simulink model "AEBWithHighFidelityDynamicsTestBench"  (R2023b)
settings: Solver=ode23tb  StartTime=0  StopTime=30  FixedStep=Ts  MaxStep=Ts  RelTol=1e-1  AbsTol=5e-3
PostLoadFcn:
  | helperSLAEBWithHighFidelityDynamicsSetup();
  | load(fullfile(matlabroot,'toolbox','driving','drivingdata','rrScenarioSimTypes.mat'));
values from neighbouring files (symbols this model uses):
  actorProfiles = helperGetActorProfiles(world.actors,OriginOffset="RearAxleCenter")    [helperSLAEBWithHighFidelityDynamicsSetup.m]
  egoActorID = id    [helperSLAEBWithHighFidelityDynamicsSetup.m]
  egoVehDyn = egoVehicleDynamicsParams(egoInitialPose, actorProfiles(egoActorID))    [helperSLAEBWithHighFidelityDynamicsSetup.m]
  m = 1575    [helperSLAEBWithHighFidelityDynamicsSetup.m]
  Ts = 0.05    [helperSLAEBWithHighFidelityDynamicsSetup.m]
  vehSim3D = repmat(     struct(         'Length', 0,         'RearOverhang', 0,         'InitialPos',[0 0 0],         'InitialRot',[0 0 0]),     numVehicles,1)    [helperSLAEBWithHighFidelityDynamicsSetup.m]
undefined symbols (not defined in the file or in its folder): Defined, Ego, Lane, maxNumActors, n, radarParams, User, v_set
libraries: roadrunnerscenario x5, simulink x4, sim3dautolib x3, sim3dprobsensorlib x2, sim3dlib x1, sim3dgroundtruthsensorlib x1, drivingsim3d x1, drivingscenarioandsensors x1
CloseFcn:
  | helperSLAEBWithHighFidelityDynamicsCleanup
settings Model: SILPILSystemUnderTest=refmodels  SnapshotInterval=5  PacingRate=0.220000  Creator=The MathWorks, Inc.  LastModifiedBy=user
settings SolverCC: MaxConsecutiveZCs=1  MaxConsecutiveMinStep=2  ZeroCrossAlgorithm=Adaptive  AlgebraicLoopSolver=TrustRegion  SolverResetMethod=Robust  MinimalZcImpactIntegration=on  MaxZcPerStep=1
settings DataIOCC: SaveOutput=off  DSMLogging=off  SaveTime=off  ReturnWorkspaceOutputs=off  Refine=3
settings OptimizationCC: DefaultParameterBehavior=Inlined  InlineInvariantSignals=on  ReuseModelBlockBuffer=off  PassReuseOutputArgsAs=Individual arguments  ZeroExternalMemoryAtStartup=off  OptimizeBlockOrder=speed  EfficientTunableParamExpr=on
settings DebuggingCC: IgnoredZcDiagnostic=none  ParameterTunabilityLossMsg=error  UnconnectedInputMsg=warning  UnconnectedOutputMsg=warning  UnconnectedLineMsg=warning  PregeneratedLibrarySubsystemCodeDiagnostic=none  ArithmeticOperatorsInVariantConditions=warning
settings HardwareCC: ProdLongLongMode=on
settings ModelReferenceCC: EnableRefExpFcnMdlSchedulingChecks=on  ModelReferenceNumInstancesAllowed=Single  PropagateVarSize=Only when enabling
settings SFSimCC: SimUseLocalCustomCode=off  CustomCodeUndefinedFunction=UseInterfaceOnly
settings RTWCC: Description=Embedded Coder  SystemTargetFile=ert.tlc  TemplateMakefile=ert_default_tmf  GenerateReport=on  RTWUseLocalCustomCode=off  Toolchain=MinGW64 | CMake/gmake (64-bit Windows)  BuildConfiguration=Release  IncludeHyperlinkInReport=on  LaunchReport=on  GenerateTraceInfo=on  GenerateTraceReport=on  GenerateTraceReportSl=on  GenerateTraceReportSf=on  GenerateTraceReportEml=on  GenerateCodeMetricsReport=on  DLArmComputeVersion=19.05
settings CodeAppCC: ForceParamTrailComments=on  IgnoreCustomStorageClasses=off  OperatorAnnotations=on  SimulinkDataObjDesc=on  SFDataObjDesc=on  CustomSymbolStrFcn=$N$M$F  InsertBlockDesc=on
settings ERTTargetCC: TargetLangStandard=C99 (ISO)  GenerateSampleERTMain=on  CombineSignalStateStructs=on  SuppressErrorStatus=on  InlinedParameterPlacement=NonHierarchical  RootIOFormat=Structure reference  RTWCAPISignals=on  ERTCustomFileTemplate=example_file_process.tlc

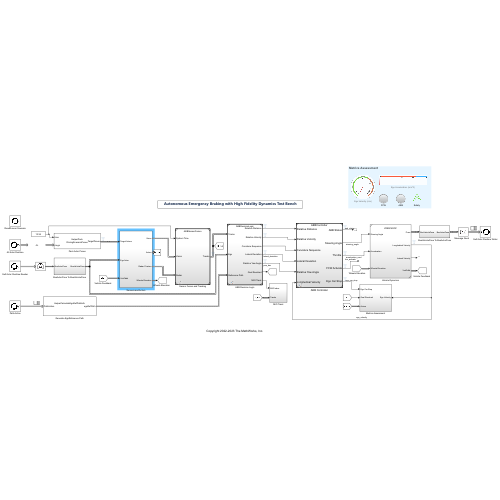
[thumbnail: Simulink's stored preview of the top-level diagram]
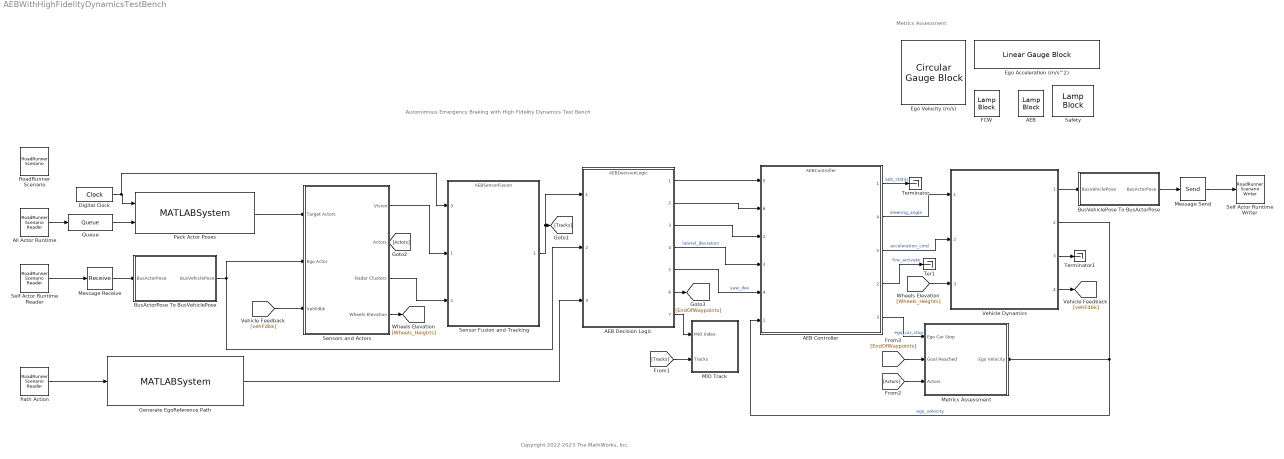
== system AEBWithHighFidelityDynamicsTestBench ==
  note: Copyright 2022-2023 The MathWorks, Inc.
  note: Autonomous Emergency Braking with High Fidelity Dynamics Test Bench
  note: Metrics Assessment
  AEB : LampBlock  LabelPosition=Hide
  AEB Controller : ModelReference  ModelNameDialog=AEBController.slx  SimulationMode=Normal  CodeInterface=Top model  ModelReferenceVersion=7.2
      settings: PortSchema="{\"entries\":[{\"content\":{\"sides\":[{\"content\":{\"connectorIds\":[\"In5\",\"In6\",\"In2\",\"In3\",\"In4\",\"In1\"]},\"type\":\"ConnectorPlacement.EquallySpacedRectSide\",\"uuid\":\"48eb62e1-c687-4ccc-af1d-5db323c86b02\"},{\"content\":{\"connectorIds\":[\"Out1\",\"Out4\",\"Out5\",\"Out2\",\"Out3\"],\"side\":\"RIGHT\"},\"type\":\"ConnectorPlacement.EquallySpacedRectSide\",\"uuid\":\"cf0b79c1-cc3c-4144-ab0a-ade48c99ebae\"},{\"content\":{\"connectorIds\":[],\"side\":\"TOP\"},\"type\":\"ConnectorPlacement.EquallySpacedRectSide\",\"uuid\":\"b5029296-17a7-4a3b-9030-50c7482e3f67\"}]},\"type\":\"ConnectorPlacement.EquallySpacedConnector\",\"uuid\":\"17fe6146-247b-40c2-bc98-b1cbe9fc8f16\"}],\"packageUris\":[\"http://schema.mathworks.com/mf0/Connector/R2020b\"],\"version\":\"1.0\"}"
  AEB Decision Logic : ModelReference  ModelNameDialog=AEBDecisionLogic.slx  SimulationMode=Normal  CodeInterface=Top model  ModelReferenceVersion=7.2
  All Actor Runtime : roadrunnerscenario/RoadRunner Scenario Reader  TopicCategory=Actor  ActorCategory=All Types  ActionType=Path Following  EventType=User-Defined  TopicType=Actor Pose (Driving Scenario compatible)  VehicleType=Vehicle Pose  UserDefinedAction=Action1  UserDefinedEvent=Event1  Filter=None  SensorTopic=Target Poses  LaneBoundaryOutputTopic=Ego-Lane  SensorID=1  SampleTime=Ts
  BusActorPose To BusVehiclePose : Subsystem
  BusVehiclePose To BusActorPose : Subsystem
  Digital Clock : DigitalClock  SampleTime=Ts
  Ego Acceleration (m/s^2) : LinearGaugeBlock  LabelPosition=Hide  ScaleMin=-9.8  ScaleMax=3  TickInterval=3
  Ego Velocity (m/s) : CircularGaugeBlock  LabelPosition=Hide  ScaleMax=25
  FCW : LampBlock  LabelPosition=Hide
  Generate EgoReference Path : MATLABSystem  InputPortMessageModes=m  System=HelperCalculateEgoRefPathInfo  EgoSpeed=v_set  SpaceResolution=DiscretizationDistance  DefaultEgoRefPath="Simulink.Bus.createMATLABStruct( \"BusEgoRefPath\" )"
      mask Type: HelperCalculateEgoRefPathInfo
      mask Display:
      | disp(['HelperCalculateEgoRefPathInfo' char(10) '' char(10) '']);
      | port_label('input',1,'PathAction');
      | port_label('output',1,'egoRefPath');
  MIO Track : Subsystem
  Message Receive : Receive  InputPortMessageModes=m  SampleTime=Ts
  "Message Send     " : Send  OutputPortMessageModes=m
  Metrics Assessment : Subsystem
      settings: PortSchema="{\"entries\":[{\"content\":{\"sides\":[{\"content\":{\"connectorIds\":[\"In1\",\"In2\",\"In3\"]},\"type\":\"ConnectorPlacement.EquallySpacedRectSide\",\"uuid\":\"d600d027-9714-4589-bd74-ff85c373770c\"},{\"content\":{\"connectorIds\":[\"In4\"],\"side\":\"RIGHT\"},\"type\":\"ConnectorPlacement.EquallySpacedRectSide\",\"uuid\":\"c68a0d3a-3a81-49cd-ba70-f2de3f1a882f\"},{\"content\":{\"connectorIds\":[],\"side\":\"TOP\"},\"type\":\"ConnectorPlacement.EquallySpacedRectSide\",\"uuid\":\"d9b15fac-7ed3-4474-96f3-d7b693286234\"},{\"content\":{\"connectorIds\":[],\"side\":\"BOTTOM\"},\"type\":\"ConnectorPlacement.EquallySpacedRectSide\",\"uuid\":\"00c5a332-b546-4dc5-aa31-259f1868ab67\"}]},\"type\":\"ConnectorPlacement.EquallySpacedConnector\",\"uuid\":\"e6d068d7-d2df-4de9-99aa-2a189a2c2730\"}],\"packageUris\":[\"http://schema.mathworks.com/mf0/Connector/R2020b\"],\"version\":\"1.0\"}"
  Pack Actor Poses : MATLABSystem  InputPortMessageModes=n,m  System=HelperPackDrivingScenarioPoses  EgoActorID=1  ActorProfiles=struct( 'ActorID', 1, 'ClassID', 1, 'Length', 4.7, 'Width', 1.8, 'Height', 1.4, 'OriginOffset', [ 0, 0, 0 ], 'FrontOverhang', 0, 'RearOverhang', 0, 'Wheelbase', 0, 'Color', [ 0, 0, 0 ] )  DefaultActorPoses="Simulink.Bus.createMATLABStruct( \"BusActors\" )"
      mask Type: HelperPackDrivingScenarioPoses
      mask Display:
      | disp(['HelperPack' char(10) 'DrivingScenarioPoses']);
      | port_label('input',1,'time');
      | port_label('input',2,'msgs');
      | port_label('output',1,'TargetPoses');
  Path Action : roadrunnerscenario/RoadRunner Scenario Reader  TopicCategory=Action  ActorCategory=All Types  ActionType=Path Following  EventType=User-Defined  TopicType=Actor Pose (Driving Scenario compatible)  VehicleType=Vehicle Specifications  UserDefinedAction=Action1  UserDefinedEvent=Event1  Filter=Self  SensorTopic=Target Poses  LaneBoundaryOutputTopic=Ego-Lane  SensorID=1  SampleTime=Ts
  Queue : Queue  InputPortMessageModes=m  OutputPortMessageModes=m  OverwriteOldest=on  Capacity=maxNumActors + 2
  RoadRunner Scenario : roadrunnerscenario/RoadRunner Scenario  UserDefinedActions={}  UserDefinedEvents={}
  Safety : LampBlock  LabelPosition=Hide  Icon=Hazards
  Self Actor Runtime Reader : roadrunnerscenario/RoadRunner Scenario Reader  TopicCategory=Actor  ActorCategory=All Types  ActionType=Path Following  EventType=User-Defined  TopicType=Actor Pose (Driving Scenario compatible)  VehicleType=Vehicle Specifications  UserDefinedAction=Action1  UserDefinedEvent=Event1  Filter=Self  SensorTopic=Target Poses  LaneBoundaryOutputTopic=Ego-Lane  SensorID=1  SampleTime=Ts
  Self Actor Runtime Writer : roadrunnerscenario/RoadRunner Scenario Writer  TopicCategory=Actor  ActorCategory=All Types  EventType=Action Complete  UserDefinedEvent=Event1  VehicleType=Vehicle Pose  TopicType=Actor Pose (Driving Scenario compatible)
  Sensor Fusion and Tracking : ModelReference  ModelNameDialog=AEBSensorFusion.slx  SimulationMode=Normal  CodeInterface=Top model  ModelReferenceVersion=7.2
      settings: PortSchema="{\"entries\":[{\"content\":{\"sides\":[{\"content\":{\"connectorIds\":[\"In3\",\"In1\",\"In2\"]},\"type\":\"ConnectorPlacement.EquallySpacedRectSide\",\"uuid\":\"d9651454-d0c0-4076-b933-d1c75ec1a64d\"},{\"content\":{\"connectorIds\":[\"Out1\"],\"side\":\"RIGHT\"},\"type\":\"ConnectorPlacement.EquallySpacedRectSide\",\"uuid\":\"0cfd8cd3-0315-45db-9435-2ff03149d1d1\"},{\"content\":{\"connectorIds\":[],\"side\":\"TOP\"},\"type\":\"ConnectorPlacement.EquallySpacedRectSide\",\"uuid\":\"cae0d945-b7aa-4a36-92d8-77152c4bc864\"}]},\"type\":\"ConnectorPlacement.EquallySpacedConnector\",\"uuid\":\"34f6be1b-6fa5-478f-9dd8-3c13b85e5ba6\"}],\"packageUris\":[\"http://schema.mathworks.com/mf0/Connector/R2020b\"],\"version\":\"1.0\"}"
  Sensors and Actors : Subsystem
  Ter1 : Terminator
  Terminator : Terminator
  Terminator1 : Terminator
  Vehicle Dynamics : Subsystem  ReferencedSubsystem=VDBS14DOF
  wires:
  AEB Controller/1 -> Terminator/1  "aeb_status"
  AEB Controller/2 -> Ter1/1  "fcw_activate"
  Vehicle Dynamics/2 -> Metrics Assessment/4(Ego Velocity), AEB Controller/1  "ego_velocity"
  [Actors] -> Metrics Assessment/3(Actors)
  [EndOfWaypoints] -> Metrics Assessment/2(Goal Reached)
  [Tracks] -> MIO Track/2(Tracks)
  AEB Controller/3 -> Metrics Assessment/1(Ego Car Stop)  "ego_car_stop"
  All Actor Runtime/1 -> Queue/1
  Queue/1 -> Pack Actor Poses/2
  Vehicle Dynamics/3 -> Terminator1/1
  Sensors and Actors/2(Actors) -> [Actors]
  Path Action/1 -> Generate EgoReference Path/1
  Pack Actor Poses/1 -> Sensors and Actors/1(Target Actors)
  AEB Controller/4 -> Vehicle Dynamics/1  "steering_angle"
  AEB Controller/5 -> Vehicle Dynamics/2  "acceleration_cmd"
  "Message Send     "/1 -> Self Actor Runtime Writer/1
  Sensors and Actors/4(Wheels Elevation) -> [Wheels_Heights]
  [vehFdbk] -> Sensors and Actors/3(VehFdbk)
  Digital Clock/1 -> Sensor Fusion and Tracking/3, Pack Actor Poses/1
  Sensor Fusion and Tracking/1 -> [Tracks], AEB Decision Logic/1
  Generate EgoReference Path/1 -> AEB Decision Logic/3
  AEB Decision Logic/6 -> [EndOfWaypoints]
  AEB Decision Logic/7 -> MIO Track/1(MIO Index)
  AEB Decision Logic/1 -> AEB Controller/5
  AEB Decision Logic/2 -> AEB Controller/6
  AEB Decision Logic/3 -> AEB Controller/2
  AEB Decision Logic/4 -> AEB Controller/3  "lateral_deviation"
  AEB Decision Logic/5 -> AEB Controller/4  "yaw_dev"
  [Wheels_Heights] -> Vehicle Dynamics/3
  Vehicle Dynamics/4 -> [vehFdbk]
  Self Actor Runtime Reader/1 -> Message Receive/1
  Message Receive/1 -> BusActorPose To BusVehiclePose/1(BusActorPose)
  BusActorPose To BusVehiclePose/1(BusVehiclePose) -> AEB Decision Logic/2, Sensors and Actors/2(Ego Actor)
  Sensors and Actors/3(Radar Clusters) -> Sensor Fusion and Tracking/2
  Sensors and Actors/1(Vision) -> Sensor Fusion and Tracking/1
  Vehicle Dynamics/1 -> BusVehiclePose To BusActorPose/1(BusVehiclePose)
  BusVehiclePose To BusActorPose/1(BusActorPose) -> "Message Send     "/1

== system AEBWithHighFidelityDynamicsTestBench/BusActorPose To BusVehiclePose ==
  BusActorPose : Inport
  Bus Creator : BusCreator  Inputs=7  OutDataTypeStr=Bus: BusVehiclePose  NonVirtualBus=on
      settings: InheritFromInputs=off
  Bus Selector : BusSelector  OutputSignals=ActorID,Position,Velocity,Roll,Pitch,Yaw,AngularVelocity
  BusVehiclePose : Outport
  wires:
  BusActorPose/1 -> Bus Selector/1
  Bus Selector/1 -> Bus Creator/1  "<ActorID>"
  Bus Selector/2 -> Bus Creator/2  "<Position>"
  Bus Selector/4 -> Bus Creator/4  "<Roll>"
  Bus Selector/5 -> Bus Creator/5  "<Pitch>"
  Bus Selector/6 -> Bus Creator/6  "<Yaw>"
  Bus Selector/7 -> Bus Creator/7  "<AngularVelocity>"
  Bus Selector/3 -> Bus Creator/3  "<Velocity>"
  Bus Creator/1 -> BusVehiclePose/1

== system AEBWithHighFidelityDynamicsTestBench/BusVehiclePose To BusActorPose ==
  BusVehiclePose : Inport
  Bus Creator : BusCreator  Inputs=7  OutDataTypeStr=Bus: BusActorPose  NonVirtualBus=on
      settings: InheritFromInputs=off
  Bus Selector : BusSelector  OutputSignals=ActorID,Position,Velocity,Roll,Pitch,Yaw,AngularVelocity
  BusActorPose : Outport
  wires:
  Bus Selector/5 -> Bus Creator/5  "<Pitch>"
  Bus Selector/1 -> Bus Creator/1  "<ActorID>"
  Bus Selector/4 -> Bus Creator/4  "<Roll>"
  Bus Selector/3 -> Bus Creator/3  "<Velocity>"
  BusVehiclePose/1 -> Bus Selector/1
  Bus Selector/6 -> Bus Creator/6  "<Yaw>"
  Bus Selector/7 -> Bus Creator/7  "<AngularVelocity>"
  Bus Selector/2 -> Bus Creator/2  "<Position>"
  Bus Creator/1 -> BusActorPose/1

== system AEBWithHighFidelityDynamicsTestBench/MIO Track ==
  note: Extract MIO and Package as Track for Visualization in Birds Eye Scope
  MIO Index : Inport
  Tracks : Inport  Port=2
  Pack MIO Track : MATLAB Function  TreatAsAtomicUnit=on
  Terminator : Terminator
  wires:
  Pack MIO Track/1(mioTrack) -> Terminator/1  "mio_track"
  Tracks/1 -> Pack MIO Track/1(tracks)
  MIO Index/1 -> Pack MIO Track/2(mioTrackIndex)

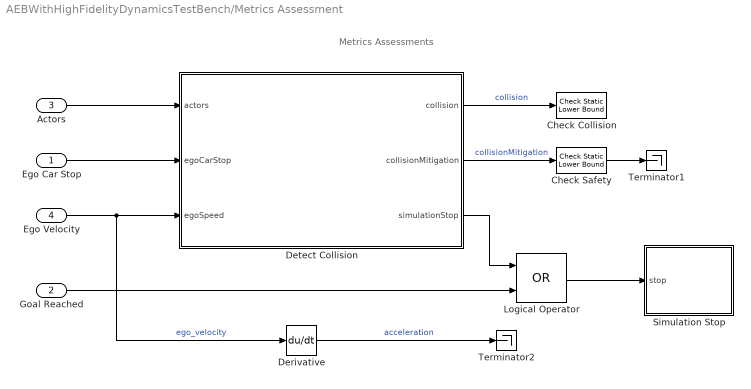
== system AEBWithHighFidelityDynamicsTestBench/Metrics Assessment ==
  note: Metrics Assessments
  Ego Car Stop : Inport
  Goal Reached : Inport  Port=2
  Actors : Inport  Port=3
  Ego Velocity : Inport  Port=4
  Check Collision : simulink/Model Verification/Check Static  Lower Bound  Description=0 <= u  min=0  min_included=on  enabled=on  stopWhenAssertionFail=off  export=off  icon=graphic
  Check Safety : simulink/Model Verification/Check Static  Lower Bound  Description=safetyGoal <= u  min=safetyGoal  min_included=on  enabled=on  stopWhenAssertionFail=off  export=on  icon=graphic
  Derivative : Derivative
  Detect Collision : MATLAB Function  TreatAsAtomicUnit=on  mask(Detect Collision){vehicleProfiles=actorProfiles, setSpeed=v_set, egoActorID=egoActorID}
      mask prompts: vehicleProfiles "Vehicle profiles"; setSpeed "Set Speed"; egoActorID "Ego Actor ID"
      mask help:
      | Detect collision between ego and target vehicles.
      | Vehicle profiles is expected to be the struture returned by the actorProfiles method of a drivingScenerio object.
      settings: AttributesFormatString=|
      | ------------------------------------------
      | vehicleProfiles = %<vehicleProfiles>
  Logical Operator : Logic  Operator=OR  AllPortsSameDT=off  OutDataTypeStr=boolean
  Simulation Stop : MATLAB Function  TreatAsAtomicUnit=on
  Terminator1 : Terminator
  Terminator2 : Terminator
  wires:
  Ego Car Stop/1 -> Detect Collision/2(egoCarStop)
  Derivative/1 -> Terminator2/1  "acceleration"
  Ego Velocity/1 -> Derivative/1, Detect Collision/3(egoSpeed)  "ego_velocity"
  Actors/1 -> Detect Collision/1(actors)
  Detect Collision/1(collision) -> Check Collision/1  "collision"
  Detect Collision/2(collisionMitigation) -> Check Safety/1  "collisionMitigation"
  Goal Reached/1 -> Logical Operator/2
  Detect Collision/3(simulationStop) -> Logical Operator/1
  Check Safety/1 -> Terminator1/1
  Logical Operator/1 -> Simulation Stop/1(stop)

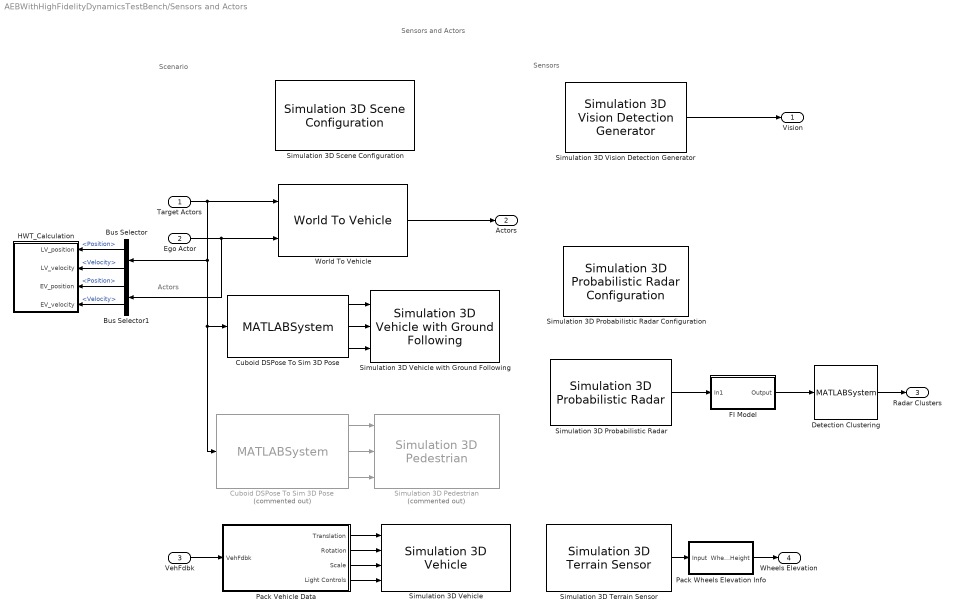
== system AEBWithHighFidelityDynamicsTestBench/Sensors and Actors ==
  note: Sensors
  note: Actors
  note: Scenario
  note: Sensors and Actors
  Target Actors : Inport
  Ego Actor : Inport  Port=2
  VehFdbk : Inport  Port=3
  Bus Selector : BusSelector  OutputSignals=Actors.Position,Actors.Velocity
  Bus Selector1 : BusSelector  OutputSignals=Position,Velocity
  Cuboid DSPose To Sim 3D Pose : MATLABSystem  System=HelperConvertDSPoseToSim3D  ActorProfiles=actorProfiles  ActorIDToConvert=2  SimulateUsing=Interpreted execution
      mask Type: HelperConvertDSPoseToSim3D
      mask Display:
      | disp(['HelperConvert' char(10) 'DSPoseToSim3D' char(10) 'ActorID: 2']);
      | port_label('input',1,'Actor');
      | port_label('output',1,'X');
      | port_label('output',2,'Y');
      | port_label('output',3,'Yaw');
  "Cuboid DSPose To Sim 3D Pose  " : MATLABSystem  Commented=on  System=HelperConvertDSPoseToSim3D  ActorProfiles=actorProfiles  ActorIDToConvert=3  SimulateUsing=Interpreted execution
      mask Type: HelperConvertDSPoseToSim3D
      mask Display:
      | disp(['HelperConvert' char(10) 'DSPoseToSim3D' char(10) 'ActorID: 3']);
      | port_label('input',1,'Actor');
      | port_label('output',1,'X');
      | port_label('output',2,'Y');
      | port_label('output',3,'Yaw');
  Detection Clustering : MATLABSystem  System=helperClusterDetections  ClusterSize=4.7  BusNameSource=Property  BusName=BusRadar  SimulateUsing=Interpreted execution
      mask Type: helperClusterDetections
      mask Display:
      | disp(['Detection' char(10) 'Clustering']);
      | port_label('input',1,'In');
      | port_label('output',1,'Out');
  FI Model : Subsystem
  HWT_Calculation : Subsystem
  Pack Vehicle Data : Subsystem
  Pack Wheels Elevation Info : Subsystem
  Simulation 3D Pedestrian : sim3dautolib/Simulation 3D Pedestrian  Priority=-1  Commented=on  PedestrianType=Male 3  Scale=[1, 1, 1]  InitialPos=vehSim3D(3).InitialPos  InitialYaw=vehSim3D(3).InitialRot  ActorName=SimulinkPedestrian1  SampleTime=-1  ActorType=SimulinkPedestrian  ActorTag=SimulinkPedestrian1  ID=1  aMode=3  CoordinateScheme=ISO  TransformOutportEnabled=off
      settings: LibrarySourceBlock=drivingsim3d/Simulation 3D Pedestrian
  Simulation 3D Probabilistic Radar : sim3dprobsensorlib/Simulation 3D Probabilistic Radar  Priority=1  sensorTag=Sim3dSensor4  sensorId=4  sensorName=Sim3dSensor4  vehTagList={'Scene Origin';'SimulinkVehicle1';'SimulinkVehicle2'}  vehTag=SimulinkVehicle1  mountLoc=Origin  offsetFlag=on  tmountOffset=radarParams.positionSim3d  rmountOffset=radarParams.rotation  AzimuthResolution=radarParams.azRes  ElevationResolution=2  RangeResolution=radarParams.rangeRes  RangeRateResolution=radarParams.rangeRateRes  AzimuthBiasFraction=0.1  ElevationBiasFraction=0.1  RangeBiasFraction=0.05  RangeRateBiasFraction=0.05  FieldOfView=[ radarParams.azFov, 5 ]  DetectionRange=radarParams.radarRange  RangeRateLimits=[ -100, 100 ]  DetectionProbability=1  FalseAlarmRate=1e-6  ReferenceRange=150  ReferenceRCS=0  HasElevation=on  HasRangeRate=on  HasNoise=off  HasFalseAlarms=off  InitialSeedSource=Repeatable  InitialSeed=0  MaxNumDetections=50  DetectionCoordinates=Sensor Cartesian  SpecifyOutputBusName=on  BusName=BusRadar  SampleTime=Ts  mountPoint=[2.424 0 0.8]  mountOrientation=[0 0 0]  aMode=3  ID=4
      settings: LibrarySourceBlock=drivingsim3d/Simulation 3D Probabilistic Radar
      settings: AttributesFormatString=|
      | -------------------------------------
      | FieldOfView = %<FieldOfView>
      | AzimuthResolution = %<AzimuthResolution>
      | DetectionCoordinates = %<DetectionCoordinates>
      | mountLoc = %<mountLoc>
      | tmountOffset = %<tmountOffset>
      | rmountOffset = %<rmountOffset>
      | Priority = %<Priority>
  Simulation 3D Probabilistic Radar Configuration : sim3dprobsensorlib/Simulation 3D Probabilistic Radar Configuration  Priority=1  RCSactorKeys=[ 4 10 7]  RCSactorProfiles={5 20 -80}  RCSdefaultValue=-20  aMode=3
      settings: LibrarySourceBlock=drivingsim3d/Simulation 3D Probabilistic Radar Configuration
  Simulation 3D Scene Configuration : sim3dlib/Simulation 3D Scene Configuration  Priority=0  ProjectFormat=RoadRunner  SceneDesc=US highway  ProjectName=C:\Program Files\MATLAB\R2023b\toolbox\shared\sim3d_projects\automotive_project_windows\UE\WindowsNoEditor\VehicleSimulation.exe  ScenePath=/Game/Maps/EmptyScene  RoadRunnerProjectPath=C:\Users\user\Desktop\roadrunner\try2311\Exports\HighwayStraightRoad.fbx  EnableOpenDRIVE=on  OpenDRIVEName=C:\RR\MyProjects\Exports\Oneteam_v1.xodr  vehTagList={'Custom';'Scene Origin';'SimulinkVehicle1';'SimulinkVehicle2'}  vehTag=SimulinkVehicle1  FreeCameraInitialTranslation=[0, 0, 0]  FreeCameraDefaultInitialTranslation=[-6, 0, 2]  FreeCameraInitialRotation=[0, 0, 0]  FreeCameraDefaultInitialRotation=[0, -15, 0]  OpVisEn=off  Ts=Ts  EnableWindow=off  EnableRemoteAccess=off  EnableWeather=off  SunAltitude=40.0  SunAzimuth=90  clouds=10  wind=1  fog=0  rain=0  EnableGeospatial=off  OriginHeight=200  OriginLatitude=40.744652  OriginLongitude=-73.988864  MapStyle=Aerial  AdditionalAssetIDs=[]  UseAdvancedSunSky=off  SolarTime=11  TimeZone=-5  Day=21  Month=9  Year=2022  UseDaylightSavingTime=on  DSTStartDay=10  DSTStartMonth=3  DSTEndDay=3  DSTEndMonth=11  DSTSwitchHour=2  sensorTag=MainCamera1  sensorId=1  sensorName=MainCamera1  mountLoc=Origin  offsetFlag=off  tmountOffset=[0, 0, 0]  rmountOffset=[0, 0, 0]  HorizontalResolution=1280  VerticalResolution=720  HorizontalFOV=60  mountPoint=[0 0 0]  mountOrientation=[0 0 0]  aMode=2  ID=1  GeoTrigger=Inactive
      settings: LibrarySourceBlock=vdynlib/Vehicle Scenarios/Sim3D/Sim3D Core/Simulation 3D Scene Configuration
  Simulation 3D Terrain Sensor : sim3dgroundtruthsensorlib/Simulation 3D Terrain Sensor  Priority=1  vehTagList={'Scene Origin';'SimulinkVehicle1'}  sensorTag=Sim3dSensor3  sensorId=3  sensorName=Sim3dSensor3  vehTag=SimulinkVehicle1  tmountOffset=[0, 0, 0]  rmountOffset=[0,0,0,]  RayOrigins=[0 0 1]  RayDirections=[0 0 -1]  RayLengths=20  NumberOfWheels=4  VisualizeTraceLines=on  SampleTime=Ts  aMode=2  ID=3
  Simulation 3D Vehicle : sim3dautolib/Simulation 3D Vehicle  Priority=-1  PassVehMesh=Sedan  MeshPath=/MathWorksSimulation/Vehicles/Muscle/Meshes/SK_MuscleCar.SK_MuscleCar  VehColor=Blue  ActorName=SimulinkVehicle1  VehLightsControl=on  HeadlightColor=[ 1, 1, 1 ]  HighBeamIntensity=100000  LowBeamIntensity=60000  HighBeamConeAngle=1.22  LowBeamConeAngle=1.22  LeftHeadlightOrientation=[ 0, 0 ]  RightHeadlightOrientation=[ 0, 0 ]  BrakelightIntensity=500  ReverselightIntensity=500  SignallightIntensity=500  SignallightPeriod=1  SignalPulseWidth=50  Translation=[egoVehDyn.X0 egoVehDyn.Y0 egoVehDyn.Z0; 0 0 0; 0 0 0; 0 0 0; 0 0 0]  Rotation=[egoVehDyn.Roll0 egoVehDyn.Pitch0 egoVehDyn.Yaw0; 0 0 0; 0 0 0; 0 0 0; 0 0 0]  Scale=ones( 5, 3 )  SampleTime=Ts  ActorType=SimulinkVehicle  ID=1  aMode=2  ActorTag=SimulinkVehicle1
  Simulation 3D Vehicle with Ground Following : sim3dautolib/Simulation 3D Vehicle with Ground Following  Priority=-1  PassVehMesh=Sedan  MeshPath=/MathWorksAutomotiveContent/Vehicles/Muscle/Meshes/SK_MuscleCar.SK_MuscleCar  TrackWidth=1.9  WheelBase=3  WheelRadius=0.35  VehColor=Red  InitialPos=vehSim3D(2).InitialPos  InitialRot=vehSim3D(2).InitialRot  ActorName=SimulinkVehicle2  SampleTime=-1  ActorType=SimulinkVehicle  ID=2  aMode=3  ActorTag=SimulinkVehicle2  CoordinateScheme=ISO  VehLightsControl=off  HeadlightColor=[ 1, 1, 1 ]  HighBeamIntensity=100000  LowBeamIntensity=60000  HighBeamConeAngle=70  LowBeamConeAngle=70  LeftHeadlightOrientation=[ 0, 0 ]  RightHeadlightOrientation=[ 0, 0 ]  BrakelightIntensity=500  ReverselightIntensity=500  SignallightIntensity=500  SignallightPeriod=1  SignalPulseWidth=50  TransformOutportEnabled=off
      settings: LibrarySourceBlock=drivingsim3d/Simulation 3D Vehicle with Ground Following
  Simulation 3D Vision Detection Generator : drivingsim3d/Simulation 3D Vision Detection Generator  Priority=1  VariantControl=Choice  sensorTag=Sim3dSensor255  sensorId=5  sensorName=Sim3dSensor2  vehTagList={'Scene Origin';'SimulinkVehicle1';'SimulinkVehicle2'}  vehTag=SimulinkVehicle1  mountLoc=Origin  offsetFlag=on  tmountOffset=cameraParams.PositionSim3d  rmountOffset=cameraParams.rotation  DetectorOutput=Objects only  MaxNumDetections=20  MaxNumLanes=30  laneSampleDistances=6:0.5:30  BusNameSource=Property  BusName=BusVision  BusName2Source=Auto  BusName2=BusVision  MaxRange=cameraParams.cameraRange  BoundingBoxAccuracy=5  ProcessNoiseIntensity=5  MaxSpeed=50  MaxAllowedOcclusion=0.5  MinObjectImageSize=[15,15]  DetectionProbability=1  FalsePositivesPerImage=0  MinLaneImageSize=[ 20, 5 ]  LaneBoundaryAccuracy=3  HasNoise=off  InitialSeedSource=Repeatable  InitialSeed=1  uniqueActorIdentifier=[]  actorClassInteger=0  cuboidLength=4.7  cuboidWidth=1.8  cuboidHeight=1.4  rotationalCenter={[-1.35, 0, 0]}  focalLength=cameraParams.focalLength  opticalCenter=cameraParams.principalPoint  imageSize=cameraParams.imageSize  radialDistortionCoefficients=[0, 0]  tangentialDistortionCoefficients=[0, 0]  cameraAxisSkew=0  actorTruthOutportEnabled=off  laneTruthOutportEnabled=off  SampleTime=Ts  checkedSampleTime=Ts  mountPoint=[0.57 0 1.2]  mountOrientation=[0 0 0]  aMode=3  ID=5
      settings: AttributesFormatString=|
      | imageSize = %<imageSize>
      | opticalCenter = %<opticalCenter>
      | focalLength = %<focalLength>
      | radialDistortionCoefficients = %<radialDistortionCoefficients>
      | mountLoc = %<mountLoc>
      | tmountOffset = %<tmountOffset>
      | rmountOffset = %<rmountOffset>
  World To Vehicle : drivingscenarioandsensors/World To Vehicle  BusNameSource=Auto  BusName=BusWorldToVehicleActors  SimulateUsing=Interpreted execution
  Vision : Outport
  Actors : Outport  Port=2
  Radar Clusters : Outport  Port=3
  Wheels Elevation : Outport  Port=4
  wires:
  Ego Actor/1 -> Bus Selector1/1, World To Vehicle/2
  Target Actors/1 -> "Cuboid DSPose To Sim 3D Pose  "/1, Cuboid DSPose To Sim 3D Pose/1, Bus Selector/1, World To Vehicle/1
  Cuboid DSPose To Sim 3D Pose/1 -> Simulation 3D Vehicle with Ground Following/1
  Cuboid DSPose To Sim 3D Pose/2 -> Simulation 3D Vehicle with Ground Following/2
  Cuboid DSPose To Sim 3D Pose/3 -> Simulation 3D Vehicle with Ground Following/3
  Pack Wheels Elevation Info/1(Wheels Height) -> Wheels Elevation/1
  World To Vehicle/1 -> Actors/1
  Detection Clustering/1 -> Radar Clusters/1
  Simulation 3D Terrain Sensor/1 -> Pack Wheels Elevation Info/1(Input)
  Pack Vehicle Data/1(Translation) -> Simulation 3D Vehicle/1
  Pack Vehicle Data/3(Scale) -> Simulation 3D Vehicle/3
  Pack Vehicle Data/2(Rotation) -> Simulation 3D Vehicle/2
  VehFdbk/1 -> Pack Vehicle Data/1(VehFdbk)
  Pack Vehicle Data/4(Light Controls) -> Simulation 3D Vehicle/4
  "Cuboid DSPose To Sim 3D Pose  "/1 -> Simulation 3D Pedestrian/1
  "Cuboid DSPose To Sim 3D Pose  "/2 -> Simulation 3D Pedestrian/2
  "Cuboid DSPose To Sim 3D Pose  "/3 -> Simulation 3D Pedestrian/3
  Simulation 3D Vision Detection Generator/1 -> Vision/1
  Simulation 3D Probabilistic Radar/1 -> FI Model/1(In1)
  FI Model/1(Output) -> Detection Clustering/1
  Bus Selector/1 -> HWT_Calculation/1(LV_position)  "<Position>"
  Bus Selector/2 -> HWT_Calculation/2(LV_velocity)  "<Velocity>"
  Bus Selector1/1 -> HWT_Calculation/3(EV_position)  "<Position>"
  Bus Selector1/2 -> HWT_Calculation/4(EV_velocity)  "<Velocity>"

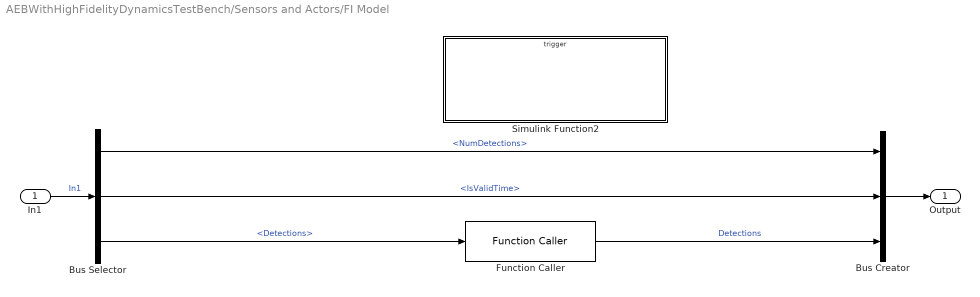
== system AEBWithHighFidelityDynamicsTestBench/Sensors and Actors/FI Model ==
  In1 : Inport
  Bus Creator : BusCreator  Inputs=3  OutDataTypeStr=Bus: BusRadar  NonVirtualBus=on
      settings: InheritFromInputs=off
  Bus Selector : BusSelector  OutputSignals=NumDetections,IsValidTime,Detections
  Function Caller : FunctionCaller  FunctionPrototype=Detections = f1(Data)  InputArgumentSpecifications=<Enter example>  OutputArgumentSpecifications=<Enter example>
  Simulink Function2 : Subsystem  TreatAsAtomicUnit=on
  Output : Outport
  wires:
  Function Caller/1 -> Bus Creator/3  "Detections"
  Bus Selector/3 -> Function Caller/1  "<Detections>"
  Bus Creator/1 -> Output/1
  Bus Selector/1 -> Bus Creator/1  "<NumDetections>"
  Bus Selector/2 -> Bus Creator/2  "<IsValidTime>"
  In1/1 -> Bus Selector/1  "In1"

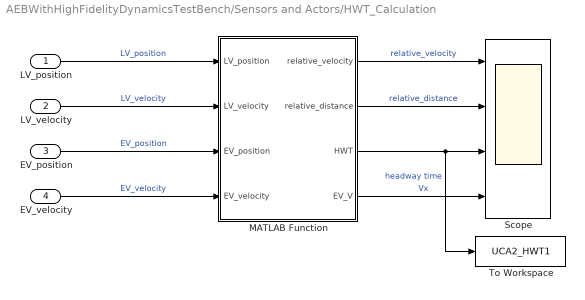
== system AEBWithHighFidelityDynamicsTestBench/Sensors and Actors/HWT_Calculation ==
  LV_position : Inport
  LV_velocity : Inport  Port=2
  EV_position : Inport  Port=3
  EV_velocity : Inport  Port=4
  MATLAB Function : MATLAB Function  TreatAsAtomicUnit=on
  Scope : Scope  NumInputPorts=4
  To Workspace : ToWorkspace  VariableName=UCA2_HWT1  SaveFormat=Timeseries  SampleTime=-1
  wires:
  LV_position/1 -> MATLAB Function/1(LV_position)  "LV_position"
  LV_velocity/1 -> MATLAB Function/2(LV_velocity)  "LV_velocity"
  EV_position/1 -> MATLAB Function/3(EV_position)  "EV_position"
  EV_velocity/1 -> MATLAB Function/4(EV_velocity)  "EV_velocity"
  MATLAB Function/1(relative_velocity) -> Scope/1  "relative_velocity"
  MATLAB Function/2(relative_distance) -> Scope/2  "relative_distance"
  MATLAB Function/3(HWT) -> To Workspace/1, Scope/3  "headway time"
  MATLAB Function/4(EV_V) -> Scope/4  "Vx"

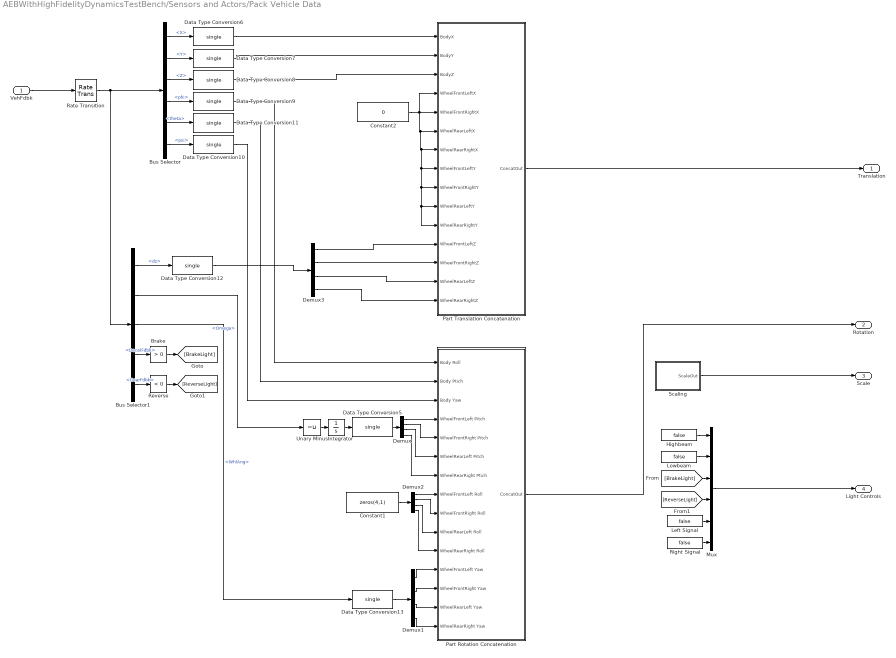
== system AEBWithHighFidelityDynamicsTestBench/Sensors and Actors/Pack Vehicle Data ==
  VehFdbk : Inport
  Brake : simulink/Logic and Bit Operations/Compare To Constant  relop=>  const=0  OutDataTypeStr=boolean  ZeroCross=off
  Bus Selector : BusSelector  OutputSignals=Body.InertFrm.Geom.Disp.X,Body.InertFrm.Geom.Disp.Y,Body.InertFrm.Geom.Disp.Z,Body.InertFrm.Cg.Ang.phi,Body.InertFrm.Cg.Ang.theta,Body.InertFrm.Cg.Ang.psi
  Bus Selector1 : BusSelector  OutputSignals=Wheels.TireFrame.dz,Wheels.TireFrame.Omega,Driveline.WhlAng,Driver.DecelFdbk,Driver.GearFdbk
  Constant1 : Constant  Value=zeros(4,1)  OutDataTypeStr=single
  Constant2 : Constant  Value=0  OutDataTypeStr=single
  Data Type Conversion{5..13} (9 alike) : DataTypeConversion  OutDataTypeStr=single  SaturateOnIntegerOverflow=off  RndMeth=Floor
  Demux{,1..3} (4 alike) : Demux
  Highbeam : Constant  Value=false
  Integrator : Integrator  WrapState=on  WrappedStateUpperValue=2*pi  WrappedStateLowerValue=0  ZeroCross=off
  Left Signal : Constant  Value=false
  Lowbeam : Constant  Value=false
  Mux : Mux  Inputs=6
  Part Rotation Concatenation : Subsystem
  Part Translation Concatenation : Subsystem
  Rate Transition : RateTransition  OutPortSampleTime=Ts
  Reverse : simulink/Logic and Bit Operations/Compare To Constant  relop=<  const=0  OutDataTypeStr=boolean  ZeroCross=off
  Right Signal : Constant  Value=false
  Scaling : Subsystem
  Unary Minus : UnaryMinus
  Translation : Outport
  Rotation : Outport  Port=2
  Scale : Outport  Port=3
  Light Controls : Outport  Port=4
  wires:
  Data Type Conversion9/1 -> Part Rotation Concatenation/1(Body Roll)
  Constant2/1 -> Part Translation Concatenation/5(WheelFrontRightX), Part Translation Concatenation/6(WheelRearLeftX), Part Translation Concatenation/7(WheelRearRightX), Part Translation Concatenation/8(WheelFrontLeftY), Part Translation Concatenation/9(WheelFrontRightY), Part Translation Concatenation/10(WheelRearLeftY), Part Translation Concatenation/11(WheelRearRightY), Part Translation Concatenation/4(WheelFrontLeftX)
  Bus Selector/5 -> Data Type Conversion11/1  "<theta>"
  Data Type Conversion6/1 -> Part Translation Concatenation/1(BodyX)
  Demux/2 -> Part Rotation Concatenation/5(WheelFrontRight Pitch)
  Constant1/1 -> Demux2/1
  Demux3/1 -> Part Translation Concatenation/12(WheelFrontLeftZ)
  Bus Selector/2 -> Data Type Conversion7/1  "<Y>"
  Bus Selector1/4 -> Brake/1  "<DecelFdbk>"
  Demux3/2 -> Part Translation Concatenation/13(WheelFrontRightZ)
  Reverse/1 -> [ReverseLight]
  Bus Selector/6 -> Data Type Conversion10/1  "<psi>"
  Demux/3 -> Part Rotation Concatenation/6(WheelRearLeft Pitch)
  Data Type Conversion11/1 -> Part Rotation Concatenation/2(Body Ptich)
  Left Signal/1 -> Mux/5
  Part Rotation Concatenation/1(ConcatOut) -> Rotation/1
  Data Type Conversion7/1 -> Part Translation Concatenation/2(BodyY)
  Rate Transition/1 -> Bus Selector/1, Bus Selector1/1
  Data Type Conversion10/1 -> Part Rotation Concatenation/3(Body Yaw)
  Demux2/4 -> Part Rotation Concatenation/11(WheelRearRight Roll)
  Unary Minus/1 -> Integrator/1
  Bus Selector/3 -> Data Type Conversion8/1  "<Z>"
  Data Type Conversion13/1 -> Demux1/1
  Demux2/3 -> Part Rotation Concatenation/10(WheelRearLeft Roll)
  Lowbeam/1 -> Mux/2
  Demux/4 -> Part Rotation Concatenation/7(WheelRearRight Ptich)
  Demux1/1 -> Part Rotation Concatenation/12(WheelFrontLeft Yaw)
  [ReverseLight] -> Mux/4
  Data Type Conversion5/1 -> Demux/1
  Bus Selector/1 -> Data Type Conversion6/1  "<X>"
  Bus Selector1/2 -> Unary Minus/1  "<Omega>"
  Demux1/3 -> Part Rotation Concatenation/14(WheelRearLeft Yaw)
  Demux3/3 -> Part Translation Concatenation/14(WheelRearLeftZ)
  VehFdbk/1 -> Rate Transition/1
  Bus Selector1/3 -> Data Type Conversion13/1  "<WhlAng>"
  Demux1/2 -> Part Rotation Concatenation/13(WheelFrontRight Yaw)
  Bus Selector1/1 -> Data Type Conversion12/1  "<dz>"
  Bus Selector/4 -> Data Type Conversion9/1  "<phi>"
  Demux/1 -> Part Rotation Concatenation/4(WheelFrontLeft Pitch)
  Demux2/2 -> Part Rotation Concatenation/9(WheelFrontRight Roll)
  Demux3/4 -> Part Translation Concatenation/15(WheelRearRightZ)
  Data Type Conversion8/1 -> Part Translation Concatenation/3(BodyZ)
  Integrator/1 -> Data Type Conversion5/1
  Demux1/4 -> Part Rotation Concatenation/15(WheelRearRight Yaw)
  Data Type Conversion12/1 -> Demux3/1
  Brake/1 -> [BrakeLight]
  Demux2/1 -> Part Rotation Concatenation/8(WheelFrontLeft Roll)
  Bus Selector1/5 -> Reverse/1  "<GearFdbk>"
  [BrakeLight] -> Mux/3
  Right Signal/1 -> Mux/6
  Highbeam/1 -> Mux/1
  Part Translation Concatenation/1(ConcatOut) -> Translation/1
  Scaling/1(ScaleOut) -> Scale/1
  Mux/1 -> Light Controls/1

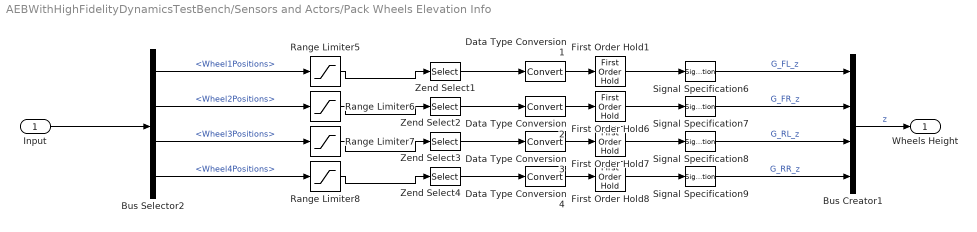
== system AEBWithHighFidelityDynamicsTestBench/Sensors and Actors/Pack Wheels Elevation Info ==
  Input : Inport
  Bus Creator1 : BusCreator  Inputs=4
  Bus Selector2 : BusSelector  OutputSignals=Wheel1Positions,Wheel2Positions,Wheel3Positions,Wheel4Positions
  Data Type Conversion{1..4} (4 alike) : DataTypeConversion  SaturateOnIntegerOverflow=off  RndMeth=Floor
  First Order Hold{1,6..8} (4 alike) : FirstOrderHold  InitialOutput=-egoVehDyn.Z0  ErrorTolerance=1
  Range Limiter{5..8} (4 alike) : Saturate  UpperLimit=1e3  LowerLimit=-1e3  ZeroCross=off
  Signal Specification{6..9} (4 alike) : SignalSpecification  Unit=m
  Zend Select{1..4} (4 alike) : Selector  NumberOfDimensions=2  InputPortWidth=3  IndexOptions=Select all,Index vector (dialog)  Indices=[1 3],3  OutputSizes=1,1
  Wheels Height : Outport
  wires:
  Range Limiter7/1 -> Zend Select3/1
  Zend Select2/1 -> Data Type Conversion2/1
  Data Type Conversion2/1 -> First Order Hold6/1
  Bus Selector2/1 -> Range Limiter5/1  "<Wheel1Positions>"
  Signal Specification7/1 -> Bus Creator1/2  "G_FR_z"
  Range Limiter8/1 -> Zend Select4/1
  Signal Specification8/1 -> Bus Creator1/3  "G_RL_z"
  Bus Selector2/2 -> Range Limiter6/1  "<Wheel2Positions>"
  First Order Hold8/1 -> Signal Specification9/1
  Bus Creator1/1 -> Wheels Height/1  "z"
  First Order Hold1/1 -> Signal Specification6/1
  Zend Select4/1 -> Data Type Conversion4/1
  Signal Specification9/1 -> Bus Creator1/4  "G_RR_z"
  Bus Selector2/3 -> Range Limiter7/1  "<Wheel3Positions>"
  Input/1 -> Bus Selector2/1
  Range Limiter6/1 -> Zend Select2/1
  Data Type Conversion3/1 -> First Order Hold7/1
  Zend Select3/1 -> Data Type Conversion3/1
  Zend Select1/1 -> Data Type Conversion1/1
  Signal Specification6/1 -> Bus Creator1/1  "G_FL_z"
  Data Type Conversion4/1 -> First Order Hold8/1
  First Order Hold7/1 -> Signal Specification8/1
  First Order Hold6/1 -> Signal Specification7/1
  Data Type Conversion1/1 -> First Order Hold1/1
  Range Limiter5/1 -> Zend Select1/1
  Bus Selector2/4 -> Range Limiter8/1  "<Wheel4Positions>"

== system AEBWithHighFidelityDynamicsTestBench/Sensors and Actors/FI Model/Simulink Function2 ==
  f1 : TriggerPort  TriggerType=function-call  IsSimulinkFunction=on  FunctionName=f1  VariantControl=(inherit)
  MATLAB Function : MATLAB Function  TreatAsAtomicUnit=on
  Simulink Function1 : Subsystem  TreatAsAtomicUnit=on
  Data : ArgIn  DisableCoverage=on  OutDataTypeStr=Bus: BusRadarDetections  PortDimensions=[50 1]  ArgumentName=Data
  Detections : ArgOut  DisableCoverage=on  OutDataTypeStr=Bus: BusRadarDetections  PortDimensions=[50 1]  ArgumentName=Detections
  wires:
  Data/1 -> MATLAB Function/1(Data)
  MATLAB Function/1(Detections) -> Detections/1

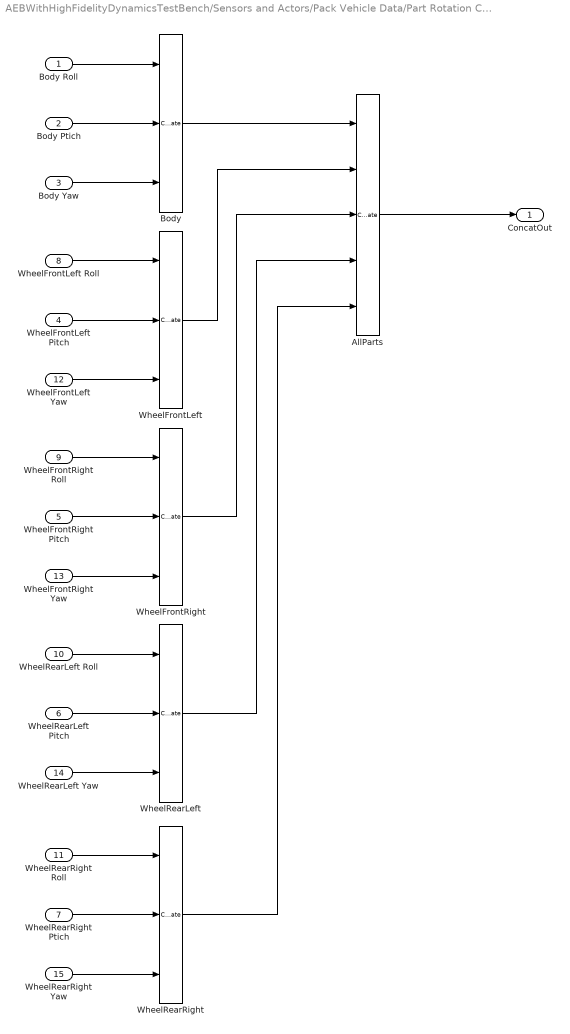
== system AEBWithHighFidelityDynamicsTestBench/Sensors and Actors/Pack Vehicle Data/Part Rotation Concatenation ==
  Body Roll : Inport
  Body Ptich : Inport  Port=2
  Body Yaw : Inport  Port=3
  WheelFrontLeft Pitch : Inport  Port=4
  WheelFrontRight Pitch : Inport  Port=5
  WheelRearLeft Pitch : Inport  Port=6
  WheelRearRight Ptich : Inport  Port=7
  WheelFrontLeft Roll : Inport  Port=8
  WheelFrontRight Roll : Inport  Port=9
  WheelRearLeft Roll : Inport  Port=10
  WheelRearRight Roll : Inport  Port=11
  WheelFrontLeft Yaw : Inport  Port=12
  WheelFrontRight Yaw : Inport  Port=13
  WheelRearLeft Yaw : Inport  Port=14
  WheelRearRight Yaw : Inport  Port=15
  AllParts : Concatenate  NumInputs=5  Mode=Multidimensional array
  Body : Concatenate  NumInputs=3  Mode=Multidimensional array  ConcatenateDimension=2
  WheelFrontLeft : Concatenate  NumInputs=3  Mode=Multidimensional array  ConcatenateDimension=2
  WheelFrontRight : Concatenate  NumInputs=3  Mode=Multidimensional array  ConcatenateDimension=2
  WheelRearLeft : Concatenate  NumInputs=3  Mode=Multidimensional array  ConcatenateDimension=2
  WheelRearRight : Concatenate  NumInputs=3  Mode=Multidimensional array  ConcatenateDimension=2
  ConcatOut : Outport  VectorParamsAs1DForOutWhenUnconnected=off
  wires:
  Body Yaw/1 -> Body/3
  WheelFrontLeft Yaw/1 -> WheelFrontLeft/3
  WheelFrontLeft/1 -> AllParts/2
  Body/1 -> AllParts/1
  WheelRearLeft/1 -> AllParts/4
  WheelFrontRight/1 -> AllParts/3
  WheelRearRight Yaw/1 -> WheelRearRight/3
  WheelRearLeft Yaw/1 -> WheelRearLeft/3
  AllParts/1 -> ConcatOut/1
  WheelRearRight/1 -> AllParts/5
  WheelFrontRight Yaw/1 -> WheelFrontRight/3
  Body Roll/1 -> Body/1
  Body Ptich/1 -> Body/2
  WheelFrontLeft Pitch/1 -> WheelFrontLeft/2
  WheelFrontLeft Roll/1 -> WheelFrontLeft/1
  WheelFrontRight Roll/1 -> WheelFrontRight/1
  WheelFrontRight Pitch/1 -> WheelFrontRight/2
  WheelRearLeft Roll/1 -> WheelRearLeft/1
  WheelRearLeft Pitch/1 -> WheelRearLeft/2
  WheelRearRight Roll/1 -> WheelRearRight/1
  WheelRearRight Ptich/1 -> WheelRearRight/2

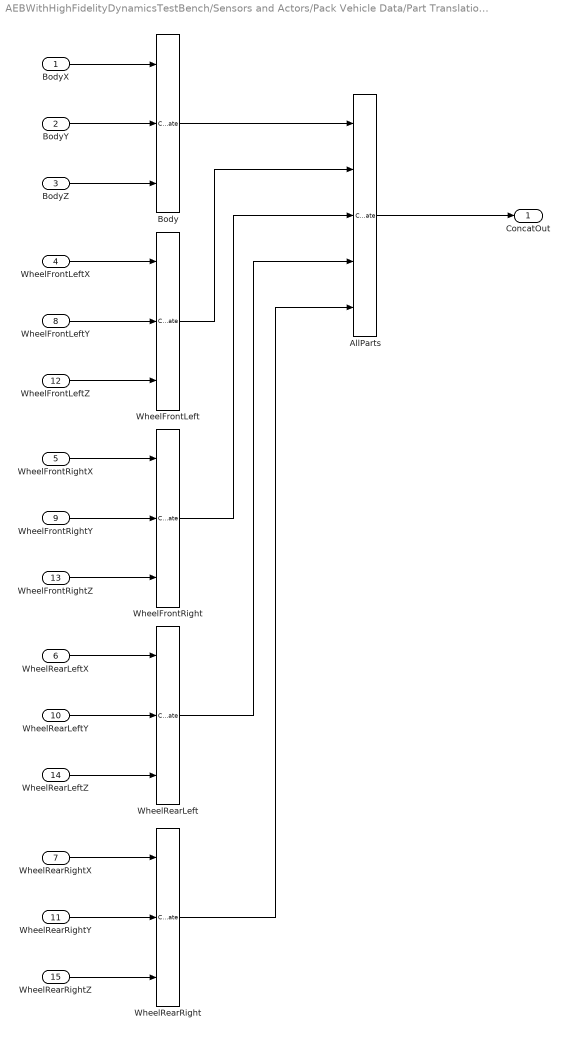
== system AEBWithHighFidelityDynamicsTestBench/Sensors and Actors/Pack Vehicle Data/Part Translation Concatenation ==
  BodyX : Inport
  BodyY : Inport  Port=2
  BodyZ : Inport  Port=3
  WheelFrontLeftX : Inport  Port=4
  WheelFrontRightX : Inport  Port=5
  WheelRearLeftX : Inport  Port=6
  WheelRearRightX : Inport  Port=7
  WheelFrontLeftY : Inport  Port=8
  WheelFrontRightY : Inport  Port=9
  WheelRearLeftY : Inport  Port=10
  WheelRearRightY : Inport  Port=11
  WheelFrontLeftZ : Inport  Port=12
  WheelFrontRightZ : Inport  Port=13
  WheelRearLeftZ : Inport  Port=14
  WheelRearRightZ : Inport  Port=15
  AllParts : Concatenate  NumInputs=5  Mode=Multidimensional array
  Body : Concatenate  NumInputs=3  Mode=Multidimensional array  ConcatenateDimension=2
  WheelFrontLeft : Concatenate  NumInputs=3  Mode=Multidimensional array  ConcatenateDimension=2
  WheelFrontRight : Concatenate  NumInputs=3  Mode=Multidimensional array  ConcatenateDimension=2
  WheelRearLeft : Concatenate  NumInputs=3  Mode=Multidimensional array  ConcatenateDimension=2
  WheelRearRight : Concatenate  NumInputs=3  Mode=Multidimensional array  ConcatenateDimension=2
  ConcatOut : Outport  VectorParamsAs1DForOutWhenUnconnected=off
  wires:
  BodyX/1 -> Body/1
  BodyZ/1 -> Body/3
  WheelFrontLeftX/1 -> WheelFrontLeft/1
  WheelFrontLeftZ/1 -> WheelFrontLeft/3
  WheelFrontLeftY/1 -> WheelFrontLeft/2
  BodyY/1 -> Body/2
  WheelFrontLeft/1 -> AllParts/2
  WheelRearRightX/1 -> WheelRearRight/1
  Body/1 -> AllParts/1
  WheelRearLeft/1 -> AllParts/4
  WheelFrontRight/1 -> AllParts/3
  WheelRearRightZ/1 -> WheelRearRight/3
  WheelFrontRightY/1 -> WheelFrontRight/2
  WheelFrontRightX/1 -> WheelFrontRight/1
  WheelRearRightY/1 -> WheelRearRight/2
  WheelRearLeftZ/1 -> WheelRearLeft/3
  AllParts/1 -> ConcatOut/1
  WheelRearLeftY/1 -> WheelRearLeft/2
  WheelRearRight/1 -> AllParts/5
  WheelRearLeftX/1 -> WheelRearLeft/1
  WheelFrontRightZ/1 -> WheelFrontRight/3

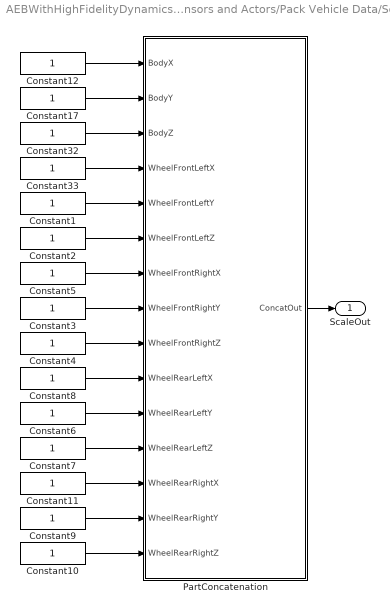
== system AEBWithHighFidelityDynamicsTestBench/Sensors and Actors/Pack Vehicle Data/Scaling ==
  Constant{1..12,17,32..33} (15 alike) : Constant  OutDataTypeStr=single
  PartConcatenation : Subsystem
  ScaleOut : Outport  VectorParamsAs1DForOutWhenUnconnected=off
  wires:
  Constant10/1 -> PartConcatenation/15(WheelRearRightZ)
  Constant9/1 -> PartConcatenation/14(WheelRearRightY)
  Constant11/1 -> PartConcatenation/13(WheelRearRightX)
  Constant7/1 -> PartConcatenation/12(WheelRearLeftZ)
  Constant6/1 -> PartConcatenation/11(WheelRearLeftY)
  Constant8/1 -> PartConcatenation/10(WheelRearLeftX)
  Constant4/1 -> PartConcatenation/9(WheelFrontRightZ)
  Constant3/1 -> PartConcatenation/8(WheelFrontRightY)
  Constant5/1 -> PartConcatenation/7(WheelFrontRightX)
  Constant2/1 -> PartConcatenation/6(WheelFrontLeftZ)
  Constant1/1 -> PartConcatenation/5(WheelFrontLeftY)
  Constant33/1 -> PartConcatenation/4(WheelFrontLeftX)
  Constant32/1 -> PartConcatenation/3(BodyZ)
  Constant17/1 -> PartConcatenation/2(BodyY)
  Constant12/1 -> PartConcatenation/1(BodyX)
  PartConcatenation/1(ConcatOut) -> ScaleOut/1

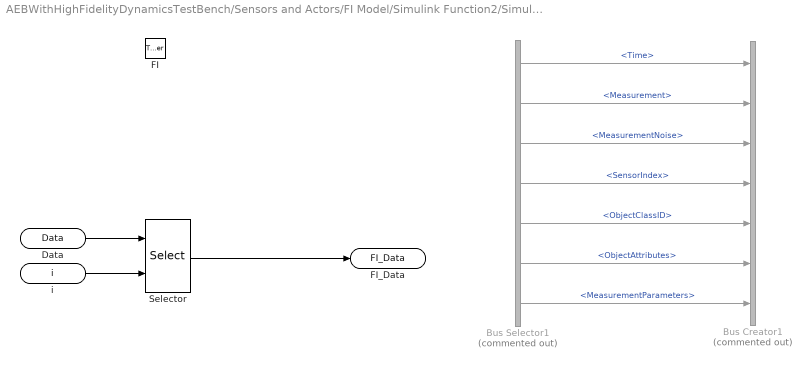
== system AEBWithHighFidelityDynamicsTestBench/Sensors and Actors/FI Model/Simulink Function2/Simulink Function1 ==
  FI : TriggerPort  TriggerType=function-call  IsSimulinkFunction=on  FunctionName=FI  FunctionVisibility=scoped  VariantControl=(inherit)
  Bus Creator1 : BusCreator  Commented=on  Inputs=7  OutDataTypeStr=Bus: BusRadarDetections  NonVirtualBus=on
  Bus Selector1 : BusSelector  Commented=on  OutputSignals=Time,Measurement,MeasurementNoise,SensorIndex,ObjectClassID,ObjectAttributes,MeasurementParameters
  Selector : Selector  InputPortWidth=50  IndexOptions=Index vector (port)  Indices=[1 3]  OutputSizes=1
  Data : ArgIn  DisableCoverage=on  OutDataTypeStr=Bus: BusRadarDetections  PortDimensions=[50 1]  ArgumentName=Data
  i : ArgIn  Port=2  ArgumentName=i
  FI_Data : ArgOut  DisableCoverage=on  OutDataTypeStr=Bus: BusRadarDetections  PortDimensions=[1 1]  ArgumentName=FI_Data
  wires:
  Bus Selector1/7 -> Bus Creator1/7  "<MeasurementParameters>"
  Bus Selector1/6 -> Bus Creator1/6  "<ObjectAttributes>"
  Bus Selector1/5 -> Bus Creator1/5  "<ObjectClassID>"
  Bus Selector1/4 -> Bus Creator1/4  "<SensorIndex>"
  Bus Selector1/3 -> Bus Creator1/3  "<MeasurementNoise>"
  Bus Selector1/2 -> Bus Creator1/2  "<Measurement>"
  Bus Selector1/1 -> Bus Creator1/1  "<Time>"
  Data/1 -> Selector/1
  i/1 -> Selector/2
  Selector/1 -> FI_Data/1

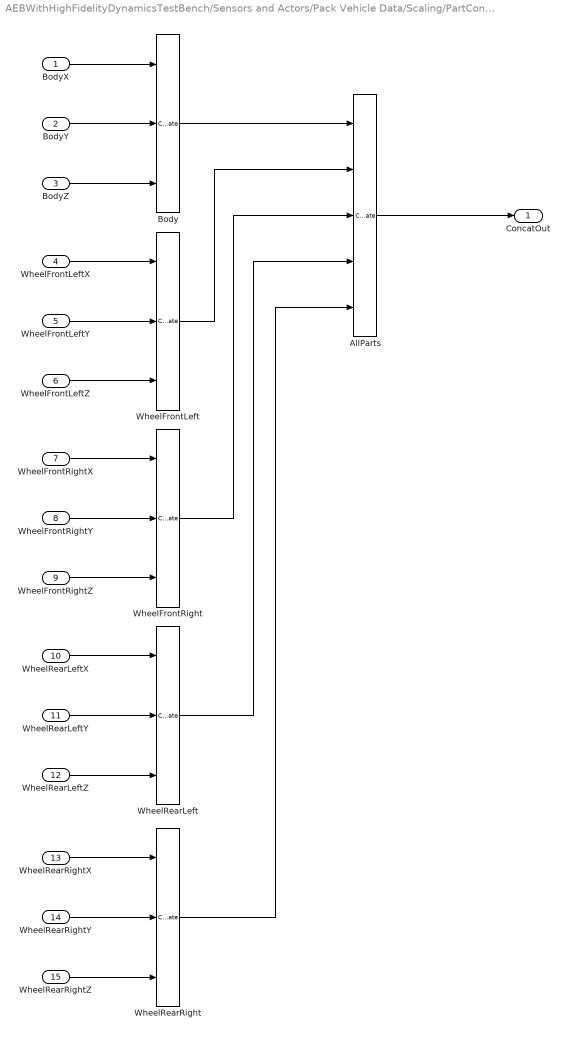
== system AEBWithHighFidelityDynamicsTestBench/Sensors and Actors/Pack Vehicle Data/Scaling/PartConcatenation ==
  BodyX : Inport
  BodyY : Inport  Port=2
  BodyZ : Inport  Port=3
  WheelFrontLeftX : Inport  Port=4
  WheelFrontLeftY : Inport  Port=5
  WheelFrontLeftZ : Inport  Port=6
  WheelFrontRightX : Inport  Port=7
  WheelFrontRightY : Inport  Port=8
  WheelFrontRightZ : Inport  Port=9
  WheelRearLeftX : Inport  Port=10
  WheelRearLeftY : Inport  Port=11
  WheelRearLeftZ : Inport  Port=12
  WheelRearRightX : Inport  Port=13
  WheelRearRightY : Inport  Port=14
  WheelRearRightZ : Inport  Port=15
  AllParts : Concatenate  NumInputs=5  Mode=Multidimensional array
  Body : Concatenate  NumInputs=3  Mode=Multidimensional array  ConcatenateDimension=2
  WheelFrontLeft : Concatenate  NumInputs=3  Mode=Multidimensional array  ConcatenateDimension=2
  WheelFrontRight : Concatenate  NumInputs=3  Mode=Multidimensional array  ConcatenateDimension=2
  WheelRearLeft : Concatenate  NumInputs=3  Mode=Multidimensional array  ConcatenateDimension=2
  WheelRearRight : Concatenate  NumInputs=3  Mode=Multidimensional array  ConcatenateDimension=2
  ConcatOut : Outport  VectorParamsAs1DForOutWhenUnconnected=off
  wires:
  BodyX/1 -> Body/1
  BodyZ/1 -> Body/3
  WheelFrontLeftX/1 -> WheelFrontLeft/1
  WheelFrontLeftZ/1 -> WheelFrontLeft/3
  WheelFrontLeftY/1 -> WheelFrontLeft/2
  BodyY/1 -> Body/2
  WheelFrontLeft/1 -> AllParts/2
  WheelRearRightX/1 -> WheelRearRight/1
  Body/1 -> AllParts/1
  WheelRearLeft/1 -> AllParts/4
  WheelFrontRight/1 -> AllParts/3
  WheelRearRightZ/1 -> WheelRearRight/3
  WheelFrontRightY/1 -> WheelFrontRight/2
  WheelFrontRightX/1 -> WheelFrontRight/1
  WheelRearRightY/1 -> WheelRearRight/2
  WheelRearLeftZ/1 -> WheelRearLeft/3
  AllParts/1 -> ConcatOut/1
  WheelRearLeftY/1 -> WheelRearLeft/2
  WheelRearRight/1 -> AllParts/5
  WheelRearLeftX/1 -> WheelRearLeft/1
  WheelFrontRightZ/1 -> WheelFrontRight/3

== matlab function AEBWithHighFidelityDynamicsTestBench/Metrics Assessment/Detect Collision ==
  data: actors input; collision output; vehicleProfiles parameter; egoCarStop input; collisionMitigation output; simulationStop output; setSpeed parameter; egoSpeed input double; egoActorID parameter
function [collision, collisionMitigation, simulationStop] = detectCollision(actors, vehicleProfiles, egoCarStop, setSpeed, egoSpeed, egoActorID)

% Associate on-path MATLAB function
coder.extrinsic('helperSLDetectVehicleCollision', 'warning');

% Assign default value to define output data type
collision = false;

% Call on-path MATLAB function
collision = helperSLDetectVehicleCollision(actors.Actors, vehicleProfiles, egoActorID = egoActorID, NumTargetActors=actors.NumActors);

if egoCarStop==true && collision==false
    collisionMitigation = 100.0; % Full collision avoidance = 100% collision migitation
elseif collision==true % collision detection
    collisionMitigation  = 100*(setSpeed-egoSpeed)/setSpeed; % calculate collision migitation
else
    collisionMitigation = 100.0; % neither collision nor ego car stop
end 

% if collision==true
%    error('Simulation stopped because of collision');
% end

if egoCarStop==true || collision==true
    simulationStop = true;
else
    simulationStop = false;
end

== matlab function AEBWithHighFidelityDynamicsTestBench/Metrics Assessment/Simulation Stop ==
  data: stop input boolean
function simStop(stop)

coder.extrinsic('helperSLTerminateSimulation');

helperSLTerminateSimulation(stop);

end

== matlab function AEBWithHighFidelityDynamicsTestBench/MIO Track/Pack MIO Track ==
  data: tracks input; mioTrack output Bus: BusMultiObjectTracker1; mioTrackIndex input
function mioTrack = fcn(tracks, mioTrackIndex)
% Extract MIO track and package for visualization in Birds Eye Scope

mioTrack = tracks;

if mioTrackIndex > 0
    % First track represents MIO
    mioTrack.NumTracks = 1;
    mioTrack.Tracks(1) = tracks.Tracks(mioTrackIndex);
else
    % No valid MIO track
    mioTrack.NumTracks = 0;
end

== matlab function AEBWithHighFidelityDynamicsTestBench/Sensors and Actors/HWT_Calculation/MATLAB Function ==
  data: LV_position input; relative_velocity output; LV_velocity input; EV_position input; EV_velocity input; relative_distance output; HWT output; EV_V output
function [relative_velocity,relative_distance,HWT,EV_V] = fcn(LV_position, LV_velocity, EV_position, EV_velocity)

EV_V=EV_velocity(1);
relative_velocity = LV_velocity(1)-EV_velocity(1);
relative_distance = LV_position(1)-EV_position(1);

HWT=relative_distance/(EV_velocity(1)+0.1);

== matlab function AEBWithHighFidelityDynamicsTestBench/Sensors and Actors/FI Model/Simulink Function2/MATLAB Function ==
  data: Data input Bus: BusRadarDetections; Detections output Bus: BusRadarDetections size=[50 1]
function Detections = fcn(Data)
    % Create a bus object with the same properties as Data
    Detections = Data;

    for i = 1:50
        % Assuming FI is a function that works with individual elements
        Detections(i) = FI(Data, i);
    end

% function Detections = fcn(Data)
% 
% all_=Data;
% for i=1:50
%     all_(i)=FI(Data,i);
% end
% Detections=all_;
% 
% end
